simulink model "simRobotControlSystem"  (R2016b)
settings: Solver=FixedStepAuto  StartTime=0.0  StopTime=inf  FixedStep=0.01  RelTol=1e-3
PostLoadFcn:
  | robotics.ros.createSimulinkBus('simRobotControlSystem','trajectory_msgs/JointTrajectory')
model workspace (MAT data in the model file):
  SL_ROS_VariableLengthArrays_MaxSizes.CommonInfo.ArrayTruncateAction = 'EmitWarning'
  SL_ROS_VariableLengthArrays_MaxSizes.MsgTypeMap = containers.Map
  SL_ROS_VariableLengthArrays_MaxSizes.MsgTypeMap.serialization.keys = {'trajectory_msgs/JointTrajectoryPoint'}
  SL_ROS_VariableLengthArrays_MaxSizes.MsgTypeMap.serialization.values{1}(1).PropertyName = 'Positions'
  SL_ROS_VariableLengthArrays_MaxSizes.MsgTypeMap.serialization.values{1}(1).DataType = 'double'
  SL_ROS_VariableLengthArrays_MaxSizes.MsgTypeMap.serialization.values{1}(1).MaxLength = 6
  SL_ROS_VariableLengthArrays_MaxSizes.MsgTypeMap.serialization.values{1}(2).PropertyName = 'Velocities'
  SL_ROS_VariableLengthArrays_MaxSizes.MsgTypeMap.serialization.values{1}(2).DataType = 'double'
  SL_ROS_VariableLengthArrays_MaxSizes.MsgTypeMap.serialization.values{1}(2).MaxLength = 6
  SL_ROS_VariableLengthArrays_MaxSizes.MsgTypeMap.serialization.values{1}(3).PropertyName = 'Accelerations'
  SL_ROS_VariableLengthArrays_MaxSizes.MsgTypeMap.serialization.values{1}(3).DataType = 'double'
  SL_ROS_VariableLengthArrays_MaxSizes.MsgTypeMap.serialization.values{1}(3).MaxLength = 6
  SL_ROS_VariableLengthArrays_MaxSizes.MsgTypeMap.serialization.values{1}(4).PropertyName = 'Effort'
  SL_ROS_VariableLengthArrays_MaxSizes.MsgTypeMap.serialization.values{1}(4).DataType = 'double'
  SL_ROS_VariableLengthArrays_MaxSizes.MsgTypeMap.serialization.values{1}(4).MaxLength = 6
  SL_ROS_VariableLengthArrays_MaxSizes.MsgTypeMap.serialization.uniformity = 0
  SL_ROS_VariableLengthArrays_MaxSizes.MsgTypeMap.serialization.keyType = 'char'
  SL_ROS_VariableLengthArrays_MaxSizes.MsgTypeMap.serialization.valueType = 'any'
libraries: robotlib x3
settings Model: Creator=PC15  LastModifiedBy=PC15

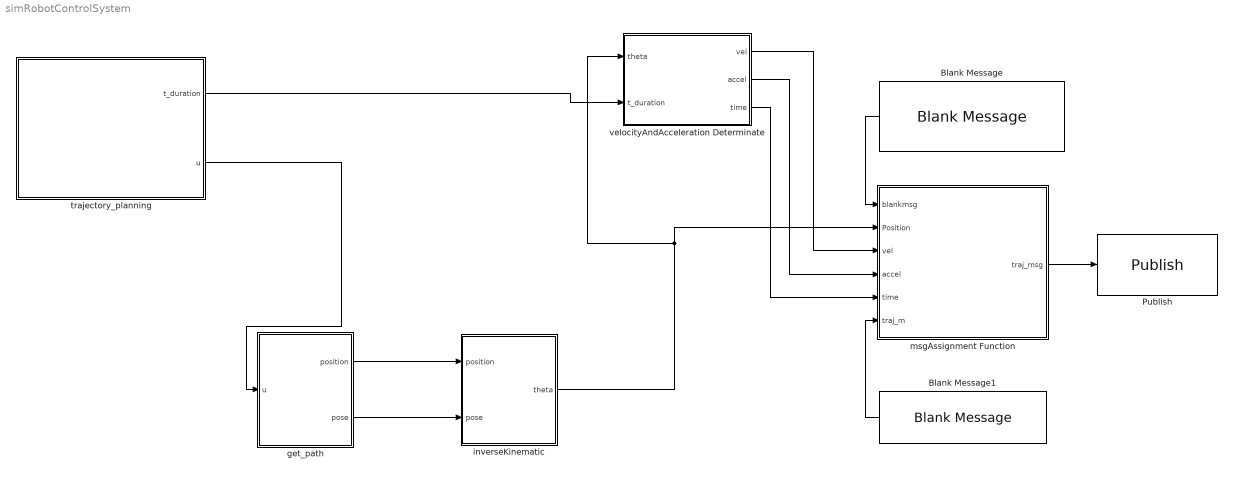
== system simRobotControlSystem ==
  Blank Message : robotlib/Blank Message  SourceLibraryInfo=This block requires Robotics System Toolbox  messageType=trajectory_msgs/JointTrajectoryPoint  SampleTime=inf
  Blank Message1 : robotlib/Blank Message  SourceLibraryInfo=This block requires Robotics System Toolbox  messageType=trajectory_msgs/JointTrajectory  SampleTime=inf
  Publish : robotlib/Publish  SourceLibraryInfo=This block requires Robotics System Toolbox  topicSource=Specify your own  topic=/trajectory_topic  messageType=trajectory_msgs/JointTrajectory  messageQueueLength=1
  get_path : MATLAB Function  TreatAsAtomicUnit=on
  inverseKinematic : MATLAB Function  TreatAsAtomicUnit=on
  msgAssignment Function : MATLAB Function  TreatAsAtomicUnit=on
  trajectory_planning : MATLAB Function  TreatAsAtomicUnit=on
  velocityAndAcceleration Determinate : MATLAB Function  TreatAsAtomicUnit=on
  wires:
  get_path/2(pose) -> inverseKinematic/2(pose)
  get_path/1(position) -> inverseKinematic/1(position)
  trajectory_planning/1(t_duration) -> velocityAndAcceleration Determinate/2(t_duration)
  Blank Message/1 -> msgAssignment Function/1(blankmsg)
  velocityAndAcceleration Determinate/2(accel) -> msgAssignment Function/4(accel)
  trajectory_planning/2(u) -> get_path/1(u)
  inverseKinematic/1(theta) -> msgAssignment Function/2(Position), velocityAndAcceleration Determinate/1(theta)
  Blank Message1/1 -> msgAssignment Function/6(traj_m)
  msgAssignment Function/1(traj_msg) -> Publish/1
  velocityAndAcceleration Determinate/1(vel) -> msgAssignment Function/3(vel)
  velocityAndAcceleration Determinate/3(time) -> msgAssignment Function/5(time)

== matlab function simRobotControlSystem/get_path ==
  data: position output; u input; pose output
function [position,pose] = path_fcn(u)

n=size(u,1);
%get position on the path
[x,y,z] = line_function1(u);
position=[x,y,z];

%get the poses on the start point and the end point
[a_s,b_s,c_s] = line_function1(0,'pose');
[a_e,b_e,c_e] = line_function1(1,'pose');
%use linear method to interpolate the poses along the path
quaternion_s = Quaternion(rpy2r([a_s,b_s,c_s]) ); %单位 deg 
quaternion_e = Quaternion(rpy2r([a_e,b_e,c_e]) ); %单位 deg

pose=zeros(3,3,n);
for i=1:n 
quatnion=interp(quaternion_s,quaternion_e,u(i));
pose(:,:,i)=quatnion.R;
end

end

== matlab function simRobotControlSystem/inverseKinematic ==
  data: position input; theta output; pose input
function theta  = inverseKinematic(position,pose)

% n=size(position,1);
% theta=zeros(n,6);
% coder.extrinsic('CreateFnc_ur5');
% coder.extrinsic('ikine');
% ur5 = CreateFnc_ur5();
% n=size(position,1);
% T=zeros(4,4,n);
% T(1:3,4,:)=position(:,1:3).';
% for i=1:n
%     T(1:3,1:3,i)=pose(:,:,i);
% end

% theta=ikine(ur5,T);

%data for testing the connection
theta=zeros(10,6);
theta(1,:)=[1.955632205574972;-2.078859169930500;-2.595912547875638;-0.266286622000264;5.625695870270549;0.899155696792604].';
theta(2,:)=[1.844798925761694;-1.961044862123725;-2.448798014502294;-0.251191436225992;5.306877694501541;0.848198919994083].';
theta(3,:)=[1.733965645948416;-1.843230554316951;-2.301683481128951;-0.236096250451719;4.988059518732531;0.797242143195561].';
theta(4,:)=[1.623132366135138;-1.725416246510176;-2.154568947755608;-0.221001064677447;4.669241342963522;0.746285366397040].';
theta(5,:)=[1.623132366135138;-1.725416246510176;-2.154568947755608;-0.221001064677447;4.669241342963522;0.746285366397040].';
theta(6,:)=[1.303063045443657;-1.385186219452159;-1.729723482378908;-0.177408700983761;3.748541110336537;0.599129380452190].';
theta(7,:)=[1.093827004565454;-1.162770500200917;-1.451992550375551;-0.148911523064348;3.146659053478561;0.502930171305862].';
theta(8,:)=[0.909452001183958;-0.966780573674288;-1.207257887858855;-0.123800732403197;2.616285585980668;0.418159651060963].';
theta(9,:)=[0.909452001183958;-0.966780573674288;-1.207257887858855;-0.123800732403197;2.616285585980668;0.418159651060963].';
theta(10,:)=[0.577993550666026;-0.614439409707951;-0.767282967055454;-0.078658731968288;1.662801535025007;0.265761643923311].';

end

== matlab function simRobotControlSystem/trajectory_planning ==
  data: t_duration output; u output
function [t_duration,u]   = trajectory_planning()

% 对归一化的参数进行S型曲线规划
steps=100;
u=zeros(steps+1,1);
t=zeros(steps+1,1);
[u,t]=SCurveBlend(@line_function1,0.35,0,0.8,0.6,1,steps);
%计算各个离散点的持续时间，最后一个点的持续时间置为0
n=size(t,1);
% t_duration=zeros(n,1);
% t_duration(1:n-1,:)=diff(t);
% t_duration(n,1)=0;

%data only use for testing
t_duration=[10;0.1;0.1;0.1;0.1;0.1;0.1;0.1;0.1;0.1];



end

== matlab function simRobotControlSystem/velocityAndAcceleration Determinate ==
  data: theta input; vel output; t_duration input; accel output; time output
function [vel,accel,time] = velAndAccel_calculation(theta,t_duration)

n_row=size(theta,1);
n_column=size(theta,2);
vel=zeros(n_row,n_column);
accel=zeros(n_row,n_column); 



%恢复t，方便梯度运算
t=zeros(n_row,1);
t(2:n_row,1)=t_duration(1:n_row-1,1);
t=cumsum(t);
time =t;
for i=1:n_column
    vel(:,i)=gradient(theta(:,i))./gradient(t);  %通过数值梯度的方法求关节速度和加速度
    accel(:,i)=gradient(vel(:,i))./gradient(t);
end

end

== matlab function simRobotControlSystem/msgAssignment Function ==
  data: blankmsg input; traj_msg output Bus: SL_Bus_simRobotControlSystem_JointTrajectory_kw48gx; Position input; vel input; accel input; time input; traj_m input
function traj_msg = trajectorymsg_JointTrajectory_assign(blankmsg,Position,vel,accel,time,traj_m)

% Assign the output message to be the same with input blank message

%the msgtype of the blockmsg is trajectory_msgs/JointTrajectoryPoint
%the msgtype of output message ie.traj_msg is trajectory_msgs/JointTrajectory
%the type of traj_msg should be configured in the Edit Data option in the
%Simulink Tab.But before this step,make sure that the command
%robotics.ros.createSimulinkBus() has been executed.It was written to the
%model postLoadFcn already.

blankmsg.Positions_SL_Info.CurrentLength=uint32(size(Position,2));
blankmsg.Velocities_SL_Info.CurrentLength=uint32( size(vel,2));
blankmsg.Accelerations_SL_Info.CurrentLength=uint32(size(accel,2));


traj_m.Points_SL_Info.CurrentLength =uint32( size(Position,1));

num_points=size(Position,1);
for i=1:num_points
blankmsg.Positions = Position(i,:).';
blankmsg.Velocities = vel(i,:).';
blankmsg.Accelerations = accel(i,:).';
blankmsg.TimeFromStart.Nsec=time(i,1)*10^6;
disp(i)
disp(time(i,1))
traj_m.Points(i)=blankmsg;
end

traj_msg=traj_m;

end
